simulink model "LQR_v9_two_separate_gyros"  (R2017b)
settings: Solver=VariableStepAuto  StartTime=0.0  StopTime=40  RelTol=1e-3
values from neighbouring files (symbols this model uses):
  A = [0 0 0 1 0 0 ... (first row only)    [LQR_PLACE_v9_sep_gryos.m]
  B = [0 0 ... (first row only)    [LQR_PLACE_v9_sep_gryos.m]
  C = [1 0 0 0 0 0 ... (first row only)    [LQR_PLACE_v9_sep_gryos.m]
  Dist_period = 50    [LQR_PLACE_v9_sep_gryos.m]
  Fd = 100    [LQR_PLACE_v9_sep_gryos.m]
  Init_cond = [ roll_angle, precession_angle1, precession_angle2, roll_rate,     precession_rate1, precession_rate2 ]    [LQR_PLACE_v9_sep_gryos.m]
  Ts = input('Enter sampling time ')    [LQR_PLACE_v9_sep_gryos.m]
  V = [0 ... (first row only)    [LQR_PLACE_v9_sep_gryos.m]
  W = [0 ... (first row only)    [LQR_PLACE_v9_sep_gryos.m]
  xNoise_mean = 0    [LQR_PLACE_v9_sep_gryos.m]
  xNoise_var = 0.01    [LQR_PLACE_v9_sep_gryos.m]
undefined symbols (not defined in the file or in its folder): K
libraries: simulink_extras x3
settings Model: Creator=daniel  LastModifiedBy=daniel

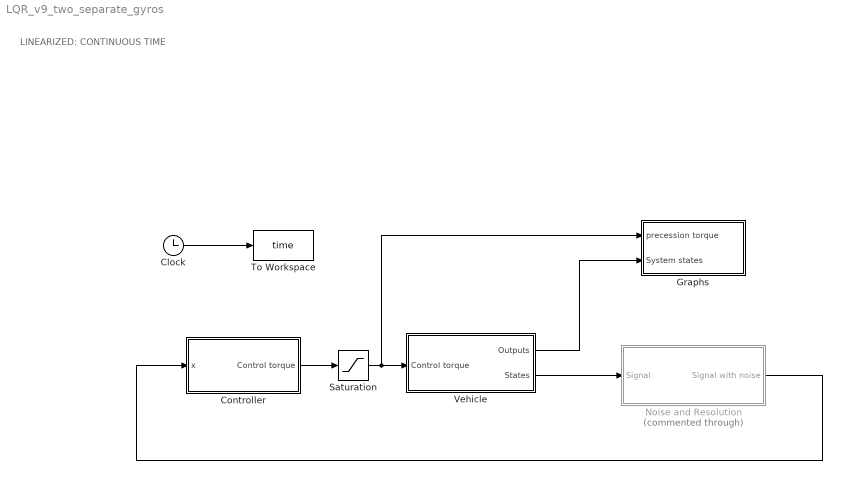
== system LQR_v9_two_separate_gyros ==
  note: LINEARIZED: CONTINUOUS TIME
  Clock : Clock
  Controller : Subsystem
  Graphs : Subsystem
  Noise and Resolution : Subsystem  Commented=through
  Saturation : Saturate  UpperLimit=70  LowerLimit=-70
  To Workspace : ToWorkspace  VariableName=time  SampleTime=-1
  "Vehicle " : Subsystem
  wires:
  Controller/1(Control torque) -> Saturation/1
  Saturation/1 -> Graphs/1(precession torque), "Vehicle "/1(Control torque)
  Clock/1 -> To Workspace/1
  "Vehicle "/1(Outputs) -> Graphs/2(System states)
  "Vehicle "/2(States) -> Noise and Resolution/1("Signal ")
  Noise and Resolution/1("Signal with noise ") -> Controller/1(x)

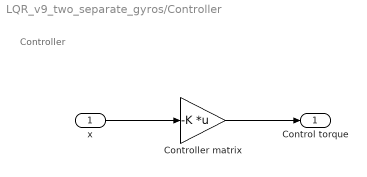
== system LQR_v9_two_separate_gyros/Controller ==
  note: Controller
  x : Inport
  Controller matrix : Gain  Gain=-K  Multiplication=Matrix(K*u)
  Control torque : Outport
  wires:
  Controller matrix/1 -> Control torque/1
  x/1 -> Controller matrix/1

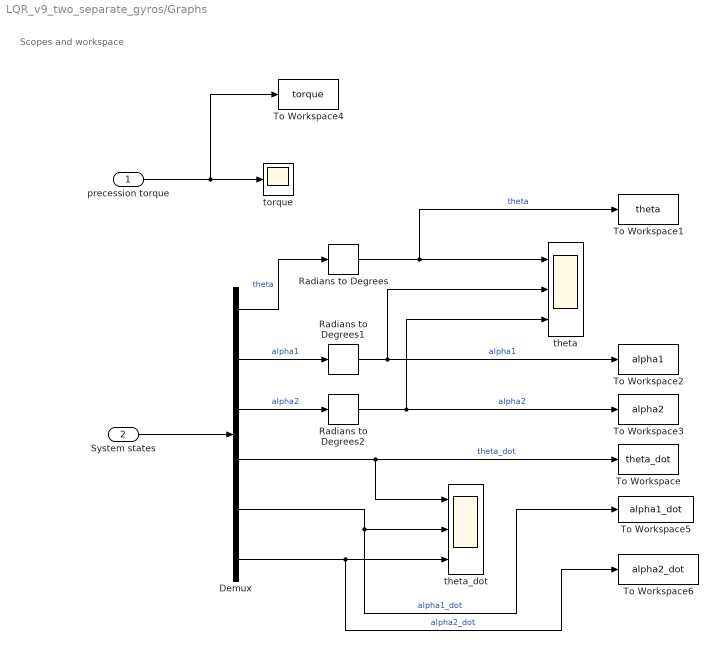
== system LQR_v9_two_separate_gyros/Graphs ==
  note: Scopes and workspace
  precession torque : Inport
  System states : Inport  Port=2
  Demux : Demux  Outputs=6
  Radians to Degrees : simulink_extras/Transformations/Radians to Degrees
  Radians to Degrees1 : simulink_extras/Transformations/Radians to Degrees
  Radians to Degrees2 : simulink_extras/Transformations/Radians to Degrees
  To Workspace : ToWorkspace  VariableName=theta_dot  SampleTime=-1
  To Workspace1 : ToWorkspace  VariableName=theta  SampleTime=-1
  To Workspace2 : ToWorkspace  VariableName=alpha1  SampleTime=-1
  To Workspace3 : ToWorkspace  VariableName=alpha2  SampleTime=-1
  To Workspace4 : ToWorkspace  VariableName=torque  SampleTime=-1
  To Workspace5 : ToWorkspace  VariableName=alpha1_dot  SampleTime=-1
  To Workspace6 : ToWorkspace  VariableName=alpha2_dot  SampleTime=-1
  theta : Scope  NumInputPorts=3
  theta_dot : Scope  NumInputPorts=3
  torque : Scope
  wires:
  System states/1 -> Demux/1
  Demux/1 -> Radians to Degrees/1  "theta"
  Demux/2 -> Radians to Degrees1/1  "alpha1"
  Demux/3 -> Radians to Degrees2/1  "alpha2"
  Demux/4 -> theta_dot/1, To Workspace/1  "theta_dot"
  Demux/5 -> theta_dot/2, To Workspace5/1  "alpha1_dot"
  Demux/6 -> To Workspace6/1, theta_dot/3  "alpha2_dot"
  Radians to Degrees1/1 -> theta/2, To Workspace2/1  "alpha1"
  Radians to Degrees/1 -> To Workspace1/1, theta/1  "theta"
  Radians to Degrees2/1 -> To Workspace3/1, theta/3  "alpha2"
  precession torque/1 -> To Workspace4/1, torque/1

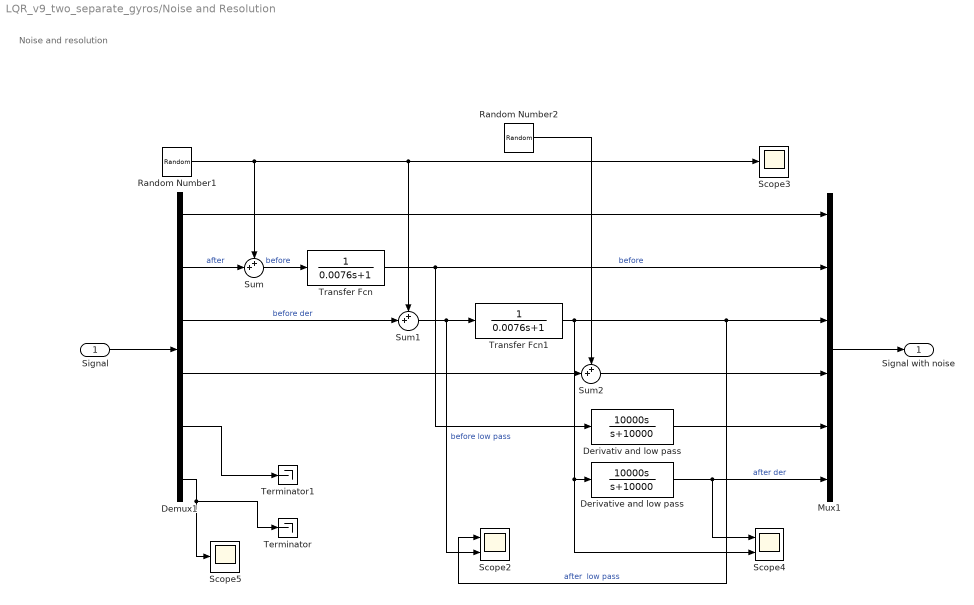
== system LQR_v9_two_separate_gyros/Noise and Resolution ==
  note: Noise and resolution
  "Signal " : Inport
  Demux1 : Demux  Outputs=6
  "Derivativ and low pass " : TransferFcn  Numerator=[10000 0]  Denominator=[1 10000]
  "Derivative and low pass " : TransferFcn  Numerator=[10000 0]  Denominator=[1 10000]
  Mux1 : Mux  Inputs=6
  Random Number1 : RandomNumber  Variance=0.00005  Seed=2345  SampleTime=0.3
  Random Number2 : RandomNumber  Variance=0.00005  Seed=2345  SampleTime=0.3
  Scope2 : Scope  NumInputPorts=2
  Scope3 : Scope
  Scope4 : Scope  NumInputPorts=2
  Scope5 : Scope
  Sum : Sum  Inputs=++|
  Sum1 : Sum  Inputs=++|
  Sum2 : Sum  Inputs=++|
  Terminator : Terminator
  Terminator1 : Terminator
  Transfer Fcn : TransferFcn  Denominator=[0.0076 1]
  Transfer Fcn1 : TransferFcn  Denominator=[0.0076 1]
  "Signal with noise " : Outport
  wires:
  Demux1/6 -> Scope5/1, Terminator/1
  Demux1/3 -> Sum1/2  "before der"
  Sum/1 -> Transfer Fcn/1  "before"
  Random Number2/1 -> Sum2/1
  Random Number1/1 -> Scope3/1, Sum1/1, Sum/1
  "Derivative and low pass "/1 -> Mux1/6, Scope4/1  "after der"
  "Derivativ and low pass "/1 -> Mux1/5
  Demux1/1 -> Mux1/1
  Sum2/1 -> Mux1/4
  Sum1/1 -> Scope2/2, Transfer Fcn1/1  "before low pass"
  Transfer Fcn/1 -> Mux1/2, "Derivativ and low pass "/1  "before"
  Demux1/2 -> Sum/2  "after"
  Demux1/5 -> Terminator1/1
  Transfer Fcn1/1 -> Scope4/2, "Derivative and low pass "/1, Mux1/3, Scope2/1  "after  low pass"
  Demux1/4 -> Sum2/2
  Mux1/1 -> "Signal with noise "/1
  "Signal "/1 -> Demux1/1

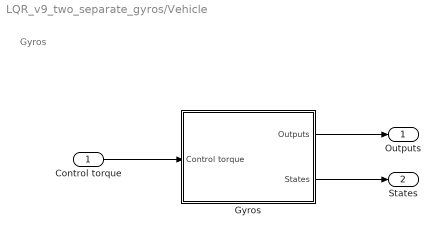
== system LQR_v9_two_separate_gyros/Vehicle  ==
  note: Gyros
  Control torque : Inport
  Gyros : Subsystem
  Outputs : Outport
  States : Outport  Port=2
  wires:
  Control torque/1 -> Gyros/1("Control torque ")
  Gyros/1(Outputs) -> Outputs/1
  Gyros/2("States ") -> States/1

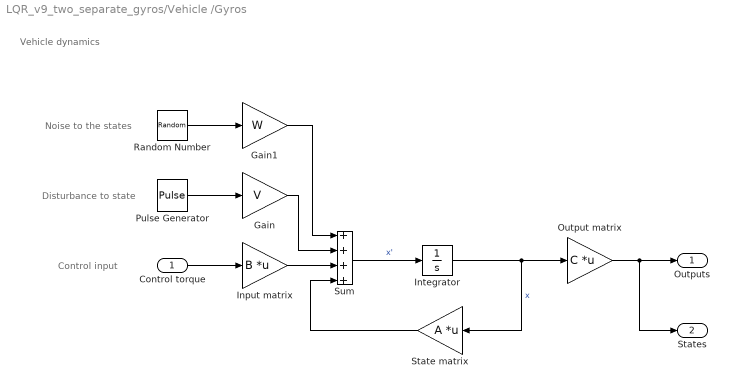
== system LQR_v9_two_separate_gyros/Vehicle /Gyros ==
  note: Noise to the states
  note: Vehicle dynamics
  note: Control input
  note: Disturbance to state
  "Control torque " : Inport
  Gain : Gain  Gain=V
  Gain1 : Gain  Gain=W
  Input matrix : Gain  Gain=B  Multiplication=Matrix(K*u)
  Integrator : Integrator  InitialCondition=Init_cond
  Output matrix : Gain  Gain=C  Multiplication=Matrix(K*u)
  Pulse Generator : DiscretePulseGenerator  PulseType=Time based  Amplitude=Fd  Period=Dist_period  PulseWidth=5  PhaseDelay=5
  Random Number : RandomNumber  Mean=xNoise_mean  Variance=xNoise_var  Seed=34567  SampleTime=Ts
  State matrix : Gain  Gain=A  Multiplication=Matrix(K*u)
  Sum : Sum  Inputs=++++
  Outputs : Outport
  "States " : Outport  Port=2
  wires:
  State matrix/1 -> Sum/4
  Output matrix/1 -> "States "/1, Outputs/1
  "Control torque "/1 -> Input matrix/1
  Sum/1 -> Integrator/1  "x'"
  Integrator/1 -> State matrix/1, Output matrix/1  "x"
  Input matrix/1 -> Sum/3
  Gain/1 -> Sum/2
  Pulse Generator/1 -> Gain/1
  Gain1/1 -> Sum/1
  Random Number/1 -> Gain1/1
